simulink model "jvd_profile"  (R2018b)
settings: Solver=FixedStepDiscrete  StartTime=0.0  StopTime=10.0  FixedStep=Ts  RelTol=1e-3
InitFcn:
  | Ts = 0.001;
libraries: peGeneralControl x3, powerlib_meascontrol x1
settings Model: Creator=Kamran  LastModifiedBy=Kamran

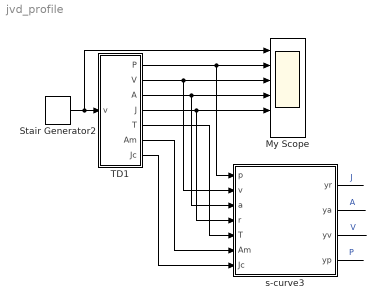
== system jvd_profile ==
  My Scope : Scope  NumInputPorts=6
  Stair Generator2 : powerlib_meascontrol/Pulse & Signal Generators/Stair Generator  t=[1, 7, 9]  e=[1, .1, 0]  Ts=Ts
      settings: SourceProductName=Simscape Power Systems
  TD1 : Subsystem  mask{x3m=3, x2m=1}
      mask prompts: x3m "x3 max"; x2m "x2 max"
  s-curve3 : MATLAB Function  TreatAsAtomicUnit=on  mask{Ps=3, D=1.5}
  wires:
  TD1/5(T) -> s-curve3/5(T)
  Stair Generator2/1 -> My Scope/1, TD1/1(v)
  TD1/3(A) -> My Scope/4, s-curve3/3(a)
  TD1/2(V) -> My Scope/3, s-curve3/2(v)
  TD1/1(P) -> s-curve3/1(p), My Scope/2
  TD1/4(J) -> My Scope/5, s-curve3/4(r)
  TD1/6(Am) -> s-curve3/6(Am)
  TD1/7(Jc) -> s-curve3/7(Jc)
  s-curve3/1(yr) -> ?  "J"
  s-curve3/2(ya) -> ?  "A"
  s-curve3/3(yv) -> ?  "V"
  s-curve3/4(yp) -> ?  "P"

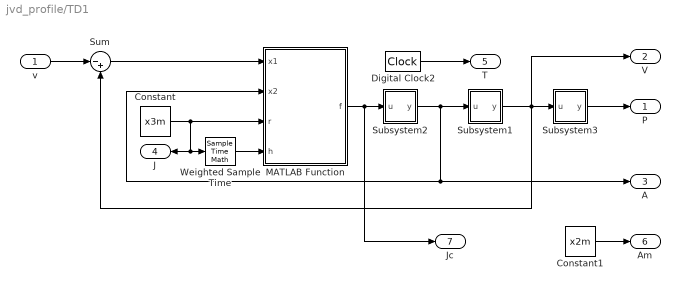
== system jvd_profile/TD1 ==
  v : Inport
  Constant : Constant  Value=x3m  SampleTime=-1
  Constant1 : Constant  Value=x2m
  Digital Clock2 : DigitalClock  SampleTime=Ts
  MATLAB Function : MATLAB Function  TreatAsAtomicUnit=on
  Subsystem1 : Subsystem  mask{sat=inf, x0=0}
      mask Display: droots([], [0], 1);
  Subsystem2 : Subsystem  mask{sat=x2m, x0=0}
      mask Display: droots([], [0], 1);
  Subsystem3 : Subsystem  mask{sat=inf, x0=0}
      mask Display: droots([], [0], 1);
  Sum : Sum  Inputs=|-+
  Weighted Sample Time : SampleTimeMath  TsampMathOp=Ts Only
  P : Outport
  V : Outport  Port=2
  A : Outport  Port=3
  J : Outport  Port=4
  T : Outport  Port=5
  Am : Outport  Port=6
  Jc : Outport  Port=7
  wires:
  Subsystem2/1(y) -> Subsystem1/1(u), A/1, MATLAB Function/2(x2)
  v/1 -> Sum/1
  Weighted Sample Time/1 -> MATLAB Function/4(h)
  Sum/1 -> MATLAB Function/1(x1)
  MATLAB Function/1(f) -> Jc/1, Subsystem2/1(u)
  Constant/1 -> J/1, Weighted Sample Time/1, MATLAB Function/3(r)
  Subsystem3/1(y) -> P/1
  Subsystem1/1(y) -> V/1, Sum/2, Subsystem3/1(u)
  Digital Clock2/1 -> T/1
  Constant1/1 -> Am/1

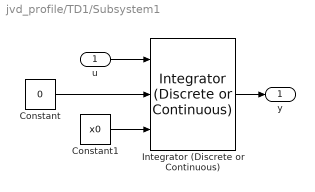
== system jvd_profile/TD1/Subsystem1 ==
  u : Inport
  Constant : Constant  Value=0
  Constant1 : Constant  Value=x0
  Integrator (Discrete or Continuous) : peGeneralControl/Integrator (Discrete or Continuous)  LabelModeActiveChoice=Discrete  ExternalReset=level  LimitType=Anti-windup  B=sat  A=-sat  Ts=-1
  y : Outport
  wires:
  Constant1/1 -> Integrator (Discrete or Continuous)/3
  u/1 -> Integrator (Discrete or Continuous)/1
  Constant/1 -> Integrator (Discrete or Continuous)/2
  Integrator (Discrete or Continuous)/1 -> y/1

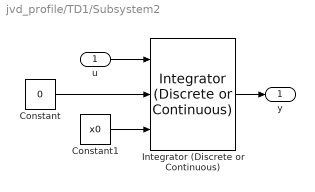
== system jvd_profile/TD1/Subsystem2 ==
  u : Inport
  Constant : Constant  Value=0
  Constant1 : Constant  Value=x0
  Integrator (Discrete or Continuous) : peGeneralControl/Integrator (Discrete or Continuous)  LabelModeActiveChoice=Discrete  ExternalReset=level  LimitType=Anti-windup  B=sat  A=-sat  Ts=-1
  y : Outport
  wires:
  Integrator (Discrete or Continuous)/1 -> y/1
  Constant/1 -> Integrator (Discrete or Continuous)/2
  u/1 -> Integrator (Discrete or Continuous)/1
  Constant1/1 -> Integrator (Discrete or Continuous)/3

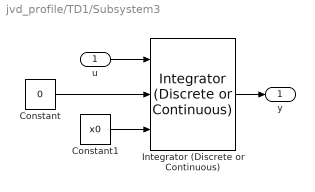
== system jvd_profile/TD1/Subsystem3 ==
  u : Inport
  Constant : Constant  Value=0
  Constant1 : Constant  Value=x0
  Integrator (Discrete or Continuous) : peGeneralControl/Integrator (Discrete or Continuous)  LabelModeActiveChoice=Discrete  ExternalReset=level  LimitType=Anti-windup  B=sat  A=-sat  Ts=-1
  y : Outport
  wires:
  Integrator (Discrete or Continuous)/1 -> y/1
  Constant/1 -> Integrator (Discrete or Continuous)/2
  u/1 -> Integrator (Discrete or Continuous)/1
  Constant1/1 -> Integrator (Discrete or Continuous)/3

== matlab function jvd_profile/s-curve3 ==
  data: yr output; Ps parameter; D parameter; p input; v input; a input; ya output; yv output; yp output; r input; T input; Am input; Jc input
function [yr, ya, yv, yp]  = profile(Ps, D,p, v, a, r, T, Am, Jc)
yr=Jc;
ya=a;
yv=v;
yp=p;
Ts=.001;
ts=4.0;
r=r*sign(Jc);

persistent t t_check t2 t_check2 Pt am jm vm dm check_change pstore vstore A;

if isempty(t);              t = 0;              end
if isempty(pstore);         pstore = 0;         end
if isempty(vstore);         vstore=0;           end
if isempty(check_change);   check_change = 0;   end
if isempty(Pt);             Pt = 0;             end
if isempty(am);             am = 0;             end
if isempty(jm);             jm = 0;             end
if isempty(vm);             vm = 0;             end
if isempty(dm);             dm = 0;             end
if isempty(t_check);        t_check = 0;        end
if isempty(t2);             t2 = 0;             end
if isempty(t_check2);       t_check2 = 0;       end
if isempty(A);              A=0;                end

if a > A
    A=a;
end
if a==Am
    t2=t2+Ts;
end

if check_change==1
    t=t+Ts;
    if Pt/vm-am/(2*jm)-vm/(2*am)-vm/(2*dm)-dm/(2*jm)>=0 && t_check-2*am/jm-vm/am+am/jm<Pt/vm-am/(2*jm)-vm/(2*am)-vm/(2*D)-D/(2*jm) 
        A=am;
        V=vm;
        J=jm;
        P=Pt;
        D=dm;

        t1 = A/J;
        t2 = V/A - A/J;
        t3 = P/V - V/(2*A)- V/(2*D) - A/(2*J)- D/(2*J);
        t4 = D/J;
        t5 = V/D - D/J;

        t = round(t / Ts) * Ts;
        t1 = round(t1 / Ts) * Ts;
        t2 = round(t2 / Ts) * Ts;
        t3 = round(t3 / Ts) * Ts;
        t4 = round(t4 / Ts) * Ts;
        t5 = round(t5 / Ts) * Ts;

        K = 2*P/(t1*(t1+t2)*(t5+2*t4+2*t3+2*t1+t2));

        if 0
        elseif t < (t1)
            yr = +K;
        elseif t < (t1 + t2)
            yr = 0;
        elseif t < (2*t1 + t2)
            yr = -K;
        elseif t < (2*t1 + t2 + t3)
            yr = 0;
        elseif t < (2*t1 + t2 + t3 + t4)
            yr = -K;
        elseif t < (2*t1 + t2 + t3 + t4 + t5)
            yr = 0;
        elseif t < (2*t1 + t2 + t3 + 2*t4 + t5)
            yr = K;
        else
            yr = 0;
        end

        if 0
        elseif t < (t1)
            ya = +K*t;
        elseif t < (t1 + t2)
            ya = +K*t1;
        elseif t < (2*t1 + t2)
            ya = +K*(2*t1+t2-t);
        elseif t < (2*t1 + t2 + t3)
            ya = 0;
        elseif t < (2*t1 + t2 + t3 + t4)
            ya = +K*(2*t1 + t2 + t3-t);
        elseif t < (2*t1 + t2 + t3 + t4 + t5)
            ya = -K*t4;
        elseif t < (2*t1 + t2 + t3 + 2*t4 + t5)
            ya = +K*(t-(2*t1 + t2 + t3 + 2*t4 + t5));
        else
            ya = 0;
        end

        if 0
        elseif t < (t1)
            yv = +K/2*t^2;
        elseif t < (t1 + t2)
            yv = +K*t1*(t-t1/2);
        elseif t < (2*t1 + t2)
            yv = +K*(-t1*t2-1*t1^2-0.5*t2^2+(2*t1+t2)*t-t^2/2);
        elseif t < (2*t1 + t2 + t3)
            yv = +K*t1*(t2+t1);
        elseif t < (2*t1 + t2 + t3 + t4)
            yv = +K*(t1*(t2+t1)-1/2*(t-2*t1-t2-t3)^2);
        elseif t < (2*t1 + t2 + t3 + t4 + t5)
            yv = +K*(t1*(t2+t1)-1/2*t4^2-t4*(t-2*t1-t2-t3-t4));
        elseif t < (2*t1 + t2 + t3 + 2*t4 + t5)
            yv = +K*(t1*(t2+t1)-t4*(t4+t5)+1/2*(t4-(t-2*t1-t2-t3-t4-t5))^2);
        else
            yv = 0;
        end

        if 0
        elseif t < (t1)
            yp = +K/6*t^3;
        elseif t < (t1 + t2)
            yp = +K*(t1^3/6+t1/2*(t-t1)*t);
        elseif t < (2*t1 + t2)
            yp = +K*(1/2*(t1^2+t1*t2)*(2*t-2*t1-t2)+(2*t1+t2-t)^3/6);
        elseif t < (2*t1 + t2 + t3)
            yp = +K/2*t1*(t2+t1)*(2*t1+t2+2*(t-2*t1-t2));
        elseif t < (2*t1 + t2 + t3 + t4)
            yp = +K*(t1/2*(t2+t1)*(2*t1+t2+2*t3+2*(t-2*t1-t2-t3))-(t-2*t1-t2-t3)^3/6);
        elseif t < (2*t1 + t2 + t3 + t4 + t5)
            yp = +K*(t1/2*(t2+t1)*(2*t1+t2+2*t3+2*t4+2*(t-2*t1-t2-t3-t4))-t4^3/6-t4^2*(t-2*t1-t2-t3-t4)/2-t4*(t-2*t1-t2-t3-t4)^2/2);
        elseif t < (2*t1 + t2 + t3 + 2*t4 + t5)
            yp = +K*(t1/2*(t2+t1)*(2*t1+t2+2*t3+2*t4+t5)-(t4-(t-2*t1-t2-t3-t4-t5))^3/6);
        else
            yp = +K*(t1/2*(t2+t1)*(2*t1+t2+2*t3+2*t4+t5)-(t4-(t4))^3/6);
        end
    else
        check_change=2;
    end
end

if(check_change==0)
    t=T;
    if ts<=t
        check_change=1;
        if a~=A && a>0 && r>0
            am=a;
            dm=D;
            jm=am^2/(2*v);
            t=am/jm;
            vm=dm^2/jm;
            Pt=Ps-p+am^3/(6*jm^2);
            if Pt/vm - vm/(2*am)- vm/(2*dm) - am/(2*jm)- dm/(2*jm)<0
                vm=(-1*(dm+am)+sqrt((dm+am)^2+8*(jm/am+jm/dm)*Pt*jm))/(2*(jm/am+jm/dm)); 
                dm=sqrt(vm*jm);
            end
        elseif a>=A
            jm=abs(r);
            am=A;
            dm=D;
            t1=am/jm;
            t2=(v-t1^2*jm/2)/(t1*jm);
            t=t2+t1;
            vm=(t2+am/jm)*am;
            Pt=Ps-p+jm*(t1^3/6+t1/2*t2^2+t1^2*t2/2);
        elseif (a~=A && a>0.0001 && r<0)
            jm=abs(r);
            am=A;
            dm=D;
            t1=am/jm;
            t=(jm*t1-a)/jm+t1+t2;
            vm=(t2+t1)*am;
            Pt=Ps-p+jm*(1/2*t1*(t2+t1)*(t2+2*(t-t2-t1))+1/6*(t1-(t-t2-t1))^3);
        elseif (a<0.0001 && a>-0.0001 && Jc<0.0001 && Jc>-0.0001)
            jm=abs(r);
            am=A;
            dm=D;
            t1=am/jm;
            vm=v;
            t2=vm/am-am/jm;
            t=(p-jm/2*t1*(t1+t2)*(2*t1+t2))/(jm*t1*(t1+t2))+2*t1+t2;
            Pt=Ps-p+jm*(1/2*t1*(t2+t1)*(2*t1+t2+2*(t-t2-2*t1)));
            t_check=t;
        end

        if vm/dm-dm/jm<0
            dm=sqrt(vm*jm);
        end
    end
end
end

== matlab function jvd_profile/TD1/MATLAB Function ==
  data: x1 input; f output; x2 input; r input; h input
function f = fhan(x1, x2, r, h)

    d = r * h^2;
    a0 = h * x2;
    y = x1 + a0;
    a1 = sqrt(d * (d + 8 * abs(y)));
    a2 = a0 + sign(y) * (a1 - d) / 2;
    sy = (sign(y + d) - sign(y - d)) / 2;
    a = (a0 + y - a2) * sy + a2;
    sa = (sign(a + d) - sign(a - d)) / 2;
    f = -r * (a / d - sign(a)) * sa - r * sign(a);
    
%     f = -sign(x1 + .5*x2*abs(x2));

end
